simulink model "Motor_Pos_Simscape"  (Simulink 7.8)
settings: Solver=ode15s  StartTime=0.0  StopTime=0.2  RelTol=1e-3
undefined symbols (not defined in the file): J, K
libraries: fl_lib x5, nesl_utility x5, elec_lib x1
settings Model: Creator=maen  LastModifiedBy=mpstme.student
settings DebuggingCC: FcnCallInpInsideContextMsg=Use local settings

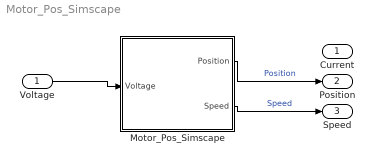
== system Motor_Pos_Simscape ==
  Voltage : Inport
  Motor_Pos_Simscape : Subsystem
  Current : Outport
  Position : Outport  Port=2
  Speed : Outport  Port=3
  wires:
  ? -> Current/1  "Current"
  Voltage/1 -> Motor_Pos_Simscape/1(Voltage)
  Motor_Pos_Simscape/1(Position) -> Position/1  "Position"
  Motor_Pos_Simscape/2(Speed) -> Speed/1  "Speed"

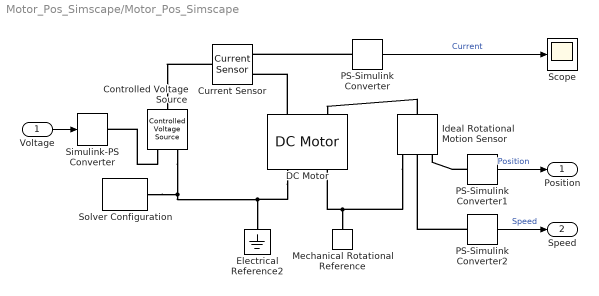
== system Motor_Pos_Simscape/Motor_Pos_Simscape ==
  Voltage : Inport
  Controlled Voltage Source : fl_lib/Electrical/Electrical Sources/Controlled Voltage Source  i_Log=off  v_Log=off  LocalVarNames=|i|v  LocalVarDescs=|i|v  LocalVarLogging=[0 0]
  Current Sensor : fl_lib/Electrical/Electrical Sensors/Current Sensor  i1_Log=off  v1_Log=off  LocalVarNames=|i1|v1  LocalVarDescs=|i1|v1  LocalVarLogging=[0 0]
  DC Motor : elec_lib/Actuators & Drivers/Rotational Actuators/DC Motor  parameterization=1  Ra=R Ohm  La=L H  emf_or_torque=1  Kv=0.0274 V/(rad/s)  Ki=K N*m/A  T_stall=2.4e-4 N*m  w_max=1.91e+4 rpm  w_rated=1.5e+4 rpm  P_rated=0.08 W  V_rated=1.5 V  J=J kg*m^2  lam_param=1  lam=b N*m/(rad/s)  i_noload=0 A  V_i_noload=1.5 V  speed0=0 rpm  current_Log=off  voltage_Log=off  power_Log=off  i2r_Log=off  torque_Log=off  speed_Log=off  LocalVarNames=|current|voltage|power|i2r|torque|speed  LocalVarDescs=|Current (A)|Voltage (V)|Power (W)|Electrical losses (W)|Torque (Nm)|Angular speed (rad/s)  LocalVarLogging=[0 0 0 0 0 0]
  Electrical Reference2 : fl_lib/Electrical/Electrical Elements/Electrical Reference  i_Log=off  LocalVarNames=|i  LocalVarDescs=|i  LocalVarLogging=[]
  Ideal Rotational Motion Sensor : fl_lib/Mechanical/Mechanical Sensors/Ideal Rotational Motion Sensor  offset=0 rad  w_Log=off  t_Log=off  phi_Log=off  LocalVarNames=|w|t|phi  LocalVarDescs=|w|t|phi  LocalVarLogging=[0 0 0]
  Mechanical Rotational Reference : fl_lib/Mechanical/Rotational Elements/Mechanical Rotational Reference  t_Log=off  LocalVarNames=|t  LocalVarDescs=|t  LocalVarLogging=0
  PS-Simulink Converter : nesl_utility/PS-Simulink Converter  PhysicalDomain=network_engine_domain  LeftPortType=input  RightPortType=output  SubClassName=ps_output  Unit=A  AffineConversion=off
  PS-Simulink Converter1 : nesl_utility/PS-Simulink Converter  PhysicalDomain=network_engine_domain  LeftPortType=input  RightPortType=output  SubClassName=ps_output  Unit=rad  AffineConversion=off
  PS-Simulink Converter2 : nesl_utility/PS-Simulink Converter  PhysicalDomain=network_engine_domain  LeftPortType=input  RightPortType=output  SubClassName=ps_output  Unit=rad/s  AffineConversion=off
  Scope : Scope
  Simulink-PS Converter : nesl_utility/Simulink-PS Converter  PhysicalDomain=network_engine_domain  LeftPortType=input  RightPortType=output  SubClassName=ps_input  Unit=V  AffineConversion=off  InputFilterTimeConstant=.001  UdotUserProvided=0
  Solver Configuration : nesl_utility/Solver Configuration  PhysicalDomain=network_engine_domain  LeftPortType=input  RightPortType=generic  SubClassName=solver  DoDC=off  ResidualTolerance=1e-9  UseLocalSolver=off  LocalSolverChoice=NE_BACKWARD_EULER_ADVANCER  LocalSolverSampleTime=.001  DoFixedCost=off  MaxNonlinIter=3  MaxModeIter=2  LinearAlgebra=Sparse  Accelerate=off  Profile=off  UseLocalSampling=off  DelaysMemoryBudget=1024
  Position : Outport
  Speed : Outport  Port=2
  wires:
  PS-Simulink Converter/1 -> Scope/1  "Current"
  PS-Simulink Converter1/1 -> Position/1  "Position"
  Voltage/1 -> Simulink-PS Converter/1
  PS-Simulink Converter2/1 -> Speed/1  "Speed"
  connections:
  Current Sensor/LConn1 -- Controlled Voltage Source/LConn1
  Controlled Voltage Source/RConn1 -- Simulink-PS Converter/RConn1
  Controlled Voltage Source/RConn2 -- DC Motor/RConn1 -- Electrical Reference2/LConn1 -- Solver Configuration/RConn1
  PS-Simulink Converter/LConn1 -- Current Sensor/RConn1
  DC Motor/LConn1 -- Current Sensor/RConn2
  Ideal Rotational Motion Sensor/LConn1 -- DC Motor/LConn2
  DC Motor/RConn2 -- Mechanical Rotational Reference/LConn1 -- Ideal Rotational Motion Sensor/RConn1
  PS-Simulink Converter2/LConn1 -- Ideal Rotational Motion Sensor/RConn2
  PS-Simulink Converter1/LConn1 -- Ideal Rotational Motion Sensor/RConn3
